simulink model "CARRIER_RECOVERY"  (R2021b)
settings: Solver=VariableStepAuto  StartTime=0.0  StopTime=0.001  RelTol=1e-3
libraries: simulink x3, dsparch4 x2, dspsigops x1, dspsrcs4 x1
settings Model: Creator=caccolillo  LastModifiedBy=caccolillo

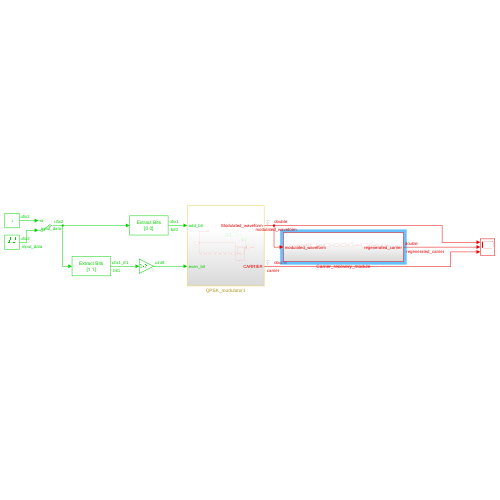
[thumbnail: Simulink's stored preview of the top-level diagram]
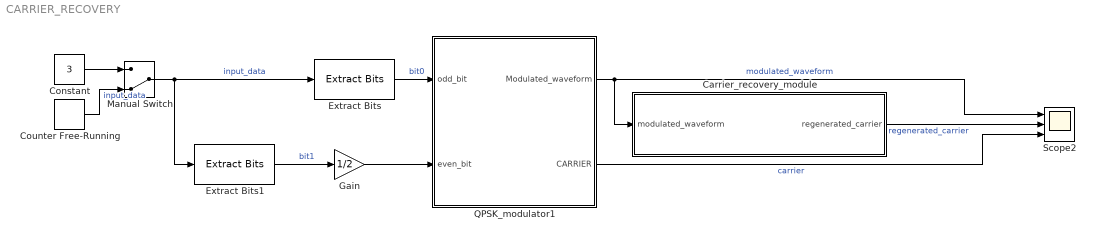
== system CARRIER_RECOVERY ==
  Carrier_recovery_module : Subsystem
  Constant : Constant  Value=3  OutDataTypeStr=fixdt(0,2)  SampleTime=1/20000
  Counter Free-Running : simulink/Sources/Counter Free-Running  NumBits=2  tsamp=1/20000
  Extract Bits : simulink/Logic and Bit Operations/Extract Bits  bitsToExtract=Range of bits  numBits=8  bitIdxRange=[0 0]  outScalingMode=Preserve fixed-point scaling
  Extract Bits1 : simulink/Logic and Bit Operations/Extract Bits  bitsToExtract=Range of bits  numBits=8  bitIdxRange=[1 1]  outScalingMode=Preserve fixed-point scaling
  Gain : Gain  Gain=1/2
  Manual Switch : ManualSwitch  CurrentSetting=0
  QPSK_modulator1 : Subsystem
  Scope2 : Scope  NumInputPorts=3
  wires:
  QPSK_modulator1/1(Modulated_waveform) -> Scope2/1, Carrier_recovery_module/1(modulated_waveform)  "modulated_waveform"
  Manual Switch/1 -> Extract Bits1/1, Extract Bits/1  "input_data"
  Gain/1 -> QPSK_modulator1/2(even_bit)
  Constant/1 -> Manual Switch/1
  Extract Bits1/1 -> Gain/1  "bit1"
  Carrier_recovery_module/1(regenerated_carrier) -> Scope2/2  "regenerated_carrier"
  Counter Free-Running/1 -> Manual Switch/2  "input_data"
  QPSK_modulator1/2(CARRIER) -> Scope2/3  "carrier"
  Extract Bits/1 -> QPSK_modulator1/1(odd_bit)  "bit0"

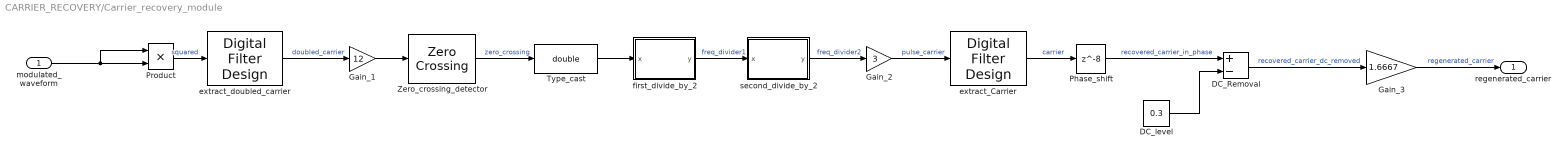
== system CARRIER_RECOVERY/Carrier_recovery_module ==
  modulated_waveform : Inport
  DC_Removal : Sum  Inputs=+-
  DC_level : Constant  Value=0.3
  Gain_1 : Gain  Gain=12
  Gain_2 : Gain  Gain=3
  Gain_3 : Gain  Gain=1.6667
  Phase_shift : Delay  DelayLength=8
  Product : Product
  Type_cast : DataTypeConversion  OutDataTypeStr=double
  Zero_crossing_detector : dspsigops/Zero Crossing  InputProcessing=Columns as channels (frame based)
      settings: SourceProductBaseCode=DS
  extract_Carrier : dsparch4/Digital Filter Design  mwdsp_browser_bugfix_var=off
  extract_doubled_carrier : dsparch4/Digital Filter Design  mwdsp_browser_bugfix_var=off
  first_divide_by_2 : MATLAB Function  TreatAsAtomicUnit=on
  second_divide_by_2 : MATLAB Function  TreatAsAtomicUnit=on
  regenerated_carrier : Outport
  wires:
  modulated_waveform/1 -> Product/1, Product/2
  DC_level/1 -> DC_Removal/2
  Gain_3/1 -> regenerated_carrier/1  "regenerated_carrier"
  Phase_shift/1 -> DC_Removal/1  "recovered_carrier_in_phase"
  DC_Removal/1 -> Gain_3/1  "recovered_carrier_dc_removed"
  Product/1 -> extract_doubled_carrier/1  "squared"
  extract_doubled_carrier/1 -> Gain_1/1  "doubled_carrier"
  Gain_2/1 -> extract_Carrier/1  "pulse_carrier"
  second_divide_by_2/1(y) -> Gain_2/1  "freq_divider2"
  first_divide_by_2/1(y) -> second_divide_by_2/1(x)  "freq_divider1"
  Gain_1/1 -> Zero_crossing_detector/1
  Type_cast/1 -> first_divide_by_2/1(x)
  extract_Carrier/1 -> Phase_shift/1  "carrier"
  Zero_crossing_detector/1 -> Type_cast/1  "zero_crossing"

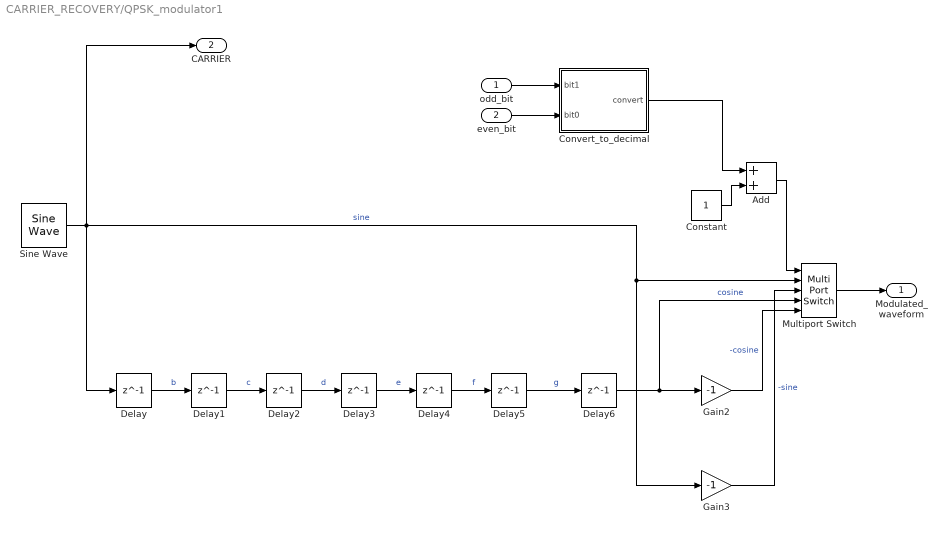
== system CARRIER_RECOVERY/QPSK_modulator1 ==
  odd_bit : Inport
  even_bit : Inport  Port=2
  Add : Sum
  Constant : Constant
  Convert_to_decimal : Subsystem
  Delay{,1..6} (7 alike) : Delay  DelayLength=1  InitialCondition=0
  Gain2 : Gain  Gain=-1
  Gain3 : Gain  Gain=-1
  Multiport Switch : MultiPortSwitch  Inputs=4
  Sine Wave : dspsrcs4/Sine Wave  Amplitude=1  Frequency=20000  Phase=0  SampleMode=Discrete  OutComplex=Real  CompMethod=Table lookup  TableSize=Speed  SampleTime=1/200000  SamplesPerFrame=1  ResetState=Restart at time zero  OutputFrames=off  dataType=double  wordLen=16  udDataType=sfix(16)  fracBitsMode=Best precision  numFracBits=15  OutDataTypeStr=double  LastOutDataTypeStr=double
  Modulated_waveform : Outport
  CARRIER : Outport  Port=2
  wires:
  Gain3/1 -> Multiport Switch/3  "-sine"
  Sine Wave/1 -> CARRIER/1, Multiport Switch/2, Gain3/1, Delay/1  "sine"
  Delay/1 -> Delay1/1  "b"
  Delay1/1 -> Delay2/1  "c"
  Delay6/1 -> Multiport Switch/4, Gain2/1  "cosine"
  Multiport Switch/1 -> Modulated_waveform/1
  Delay3/1 -> Delay4/1  "e"
  Gain2/1 -> Multiport Switch/5  "-cosine"
  Delay4/1 -> Delay5/1  "f"
  odd_bit/1 -> Convert_to_decimal/1(bit1)
  Delay2/1 -> Delay3/1  "d"
  Convert_to_decimal/1(convert) -> Add/1
  Constant/1 -> Add/2
  Add/1 -> Multiport Switch/1
  even_bit/1 -> Convert_to_decimal/2(bit0)
  Delay5/1 -> Delay6/1  "g"

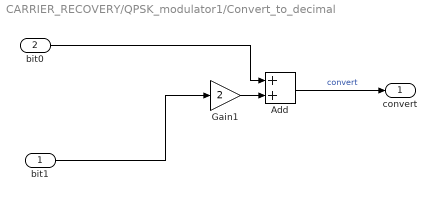
== system CARRIER_RECOVERY/QPSK_modulator1/Convert_to_decimal ==
  bit1 : Inport
  bit0 : Inport  Port=2
  Add : Sum
  Gain1 : Gain  Gain=2
  convert : Outport
  wires:
  bit1/1 -> Gain1/1
  bit0/1 -> Add/1
  Add/1 -> convert/1  "convert"
  Gain1/1 -> Add/2

== matlab function CARRIER_RECOVERY/Carrier_recovery_module/second_divide_by_2 ==
  data: x input; y output
function y = freqDivider(x)
% freqDivider  Frequency divider using persistent 2-sample input buffer
%
%   y = freqDivider(x) processes a single input sample x (scalar), and
%   returns a scalar output y, which goes high on every second rising edge.
%
%   This function is stateful and maintains internal buffer and edge counter
%   across calls using persistent variables.

    % Declare persistent variables
    persistent buf riseCount

    % Initialize persistent variables on first call
    if isempty(buf)
        buf = [0, 0];      % input buffer: [x(i-2), x(i-1)]
        riseCount = 0;     % rising edge counter
    end

    % Shift input buffer
    buf = [buf(2), x];

    % Default output
    y = 0;

    % Detect rising edge: x(i-1) <= 0 and x(i) > 0
    if buf(1) <= 0 && buf(2) > 0
        riseCount = riseCount + 1;

        if mod(riseCount, 2) == 0
            y = 1;  % Output high on every 2nd rising edge
        end
    end
end

== matlab function CARRIER_RECOVERY/Carrier_recovery_module/first_divide_by_2 ==
  data: x input; y output
function y = freqDivider(x)
% freqDivider  Frequency divider using persistent 2-sample input buffer
%
%   y = freqDivider(x) processes a single input sample x (scalar), and
%   returns a scalar output y, which goes high on every second rising edge.
%
%   This function is stateful and maintains internal buffer and edge counter
%   across calls using persistent variables.

    % Declare persistent variables
    persistent buf riseCount

    % Initialize persistent variables on first call
    if isempty(buf)
        buf = [0, 0];      % input buffer: [x(i-2), x(i-1)]
        riseCount = 0;     % rising edge counter
    end

    % Shift input buffer
    buf = [buf(2), x];

    % Default output
    y = 0;

    % Detect rising edge: x(i-1) <= 0 and x(i) > 0
    if buf(1) <= 0 && buf(2) > 0
        riseCount = riseCount + 1;

        if mod(riseCount, 2) == 0
            y = 1;  % Output high on every 2nd rising edge
        end
    end
end
